simulink model "reactive_power_compensation"  (R2017b)
settings: Solver=VariableStepAuto  StartTime=0.0  StopTime=1  MaxStep=1e-4  RelTol=1e-3
undefined symbols (not defined in the file): magnitude
libraries: powerlib x15, powerlib_meascontrol x2
settings Model: Creator=Damla  LastModifiedBy=dagac

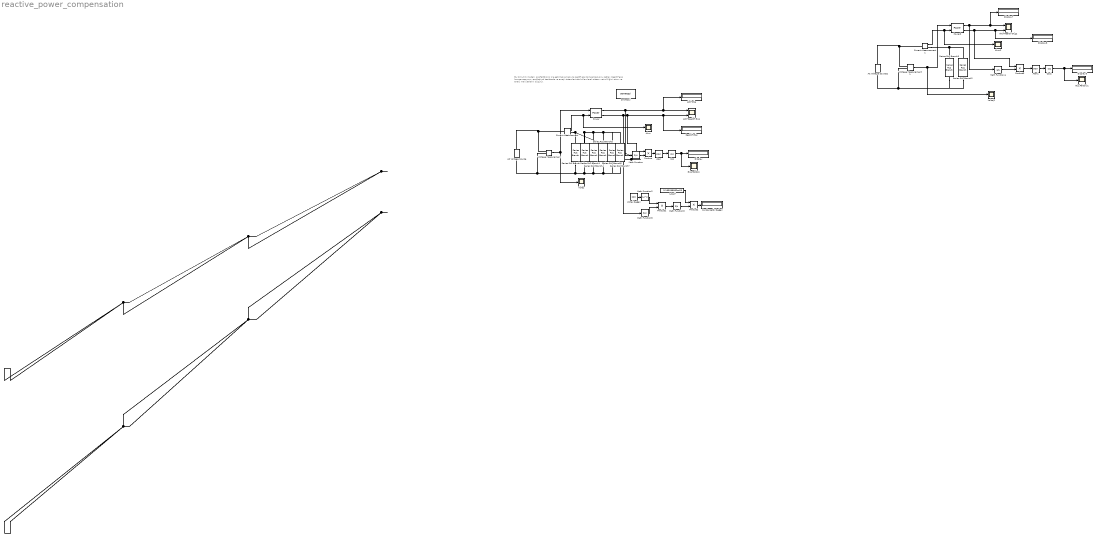
== system reactive_power_compensation ==
  note: Bu Simulink modeli, güç faktörünü 1'e getirmek amacıyla reaktif güç kompanzasyonu sağlar.
      | Reaktif güç kompanzasyonu, endüstriyel tesislerde ve enerji sistemlerinde kullanılarak
      | sistem verimliliğini artırır ve enerji maliyetlerini düşürür.
  1/2pif : Constant  Value=3.183098862e-03
  AC Voltage Source : powerlib/Electrical Sources/AC Voltage Source  Amplitude=220  Phase=0  Frequency=50  SampleTime=0  Measurements=None  BusType=swing  Pref=10e3  Qref=0  Qmin=-inf  Qmax=+inf
  AC Voltage Source2 : powerlib/Electrical Sources/AC Voltage Source  Amplitude=220  Phase=0  Frequency=50  SampleTime=0  Measurements=None  BusType=swing  Pref=10e3  Qref=0  Qmin=-inf  Qmax=+inf
  Aktif Güç : Display
  Aktif Reaktif Güç : Scope  NumInputPorts=2
  Aktif Reaktif Güç2 : Scope  NumInputPorts=2
  Akım : Scope
  Akım2 : Scope
  Atan : Trigonometry  Operator=atan
  Atan1 : Trigonometry  Operator=atan
  Cos : Trigonometry  Operator=cos
  Cos2 : Trigonometry  Operator=cos
  Current Measurement : powerlib/Measurements/Current Measurement  PhasorSimulation=off  OutputType=Complex  PSBequivalent=0
  Current Measurement1 : powerlib/Measurements/Current Measurement  PhasorSimulation=off  OutputType=Complex  PSBequivalent=0
  Display{,5,7..8} (4 alike) : Display
  Güç Faktörü : Scope
  Güç Faktörü1 : Scope
  Kondansatör Değeri : Display
  Math Function{,3..5} (4 alike) : Math  Operator=reciprocal  SaturateOnIntegerOverflow=on
  Math Function2 : Math  Operator=magnitude^2  SaturateOnIntegerOverflow=on
  Power : powerlib_meascontrol/Measurements/Power  Freq=50  Vinit=[1, 0]  Iinit=[1, 0]  Ts=0
      settings: SourceProductName=Simscape Power Systems
  Power2 : powerlib_meascontrol/Measurements/Power  Freq=50  Vinit=[1, 0]  Iinit=[1, 0]  Ts=0
      settings: SourceProductName=Simscape Power Systems
  Product{,1..3} (4 alike) : Product
  Reaktif Güç : Display
  Series RLC Branch : powerlib/Elements/Series RLC Branch  LConnTagsString=__new0  RConnTagsString=__new0  BranchType=RL  Resistance=12  Inductance=0.01  SetiL0=off  InitialCurrent=0  Capacitance=1e-6  Setx0=off  InitialVoltage=0  Measurements=None
  Series RLC Branch1 : powerlib/Elements/Series RLC Branch  LConnTagsString=__new0  RConnTagsString=__new0  BranchType=RC  Resistance=0.1  Inductance=0.01  SetiL0=off  InitialCurrent=0  Capacitance=3.25e-05  Setx0=off  InitialVoltage=0  Measurements=None
  Series RLC Branch2 : powerlib/Elements/Series RLC Branch  LConnTagsString=__new0  RConnTagsString=__new0  BranchType=RC  Resistance=0.1  Inductance=0.01  SetiL0=off  InitialCurrent=0  Capacitance=3.25e-05  Setx0=off  InitialVoltage=0  Measurements=None
  Series RLC Branch3 : powerlib/Elements/Series RLC Branch  LConnTagsString=__new0  RConnTagsString=__new0  BranchType=RL  Resistance=12  Inductance=0.01  SetiL0=off  InitialCurrent=0  Capacitance=1e-6  Setx0=off  InitialVoltage=0  Measurements=None
  Series RLC Branch4 : powerlib/Elements/Series RLC Branch  LConnTagsString=__new0  RConnTagsString=__new0  BranchType=RC  Resistance=0.1  Inductance=0.01  SetiL0=off  InitialCurrent=0  Capacitance=1.624e-05  Setx0=off  InitialVoltage=0  Measurements=None
  Series RLC Branch5 : powerlib/Elements/Series RLC Branch  LConnTagsString=__new0  RConnTagsString=__new0  BranchType=RC  Resistance=0.1  Inductance=0.01  SetiL0=off  InitialCurrent=0  Capacitance=8.124e-06  Setx0=off  InitialVoltage=0  Measurements=None
  Series RLC Branch6 : powerlib/Elements/Series RLC Branch  LConnTagsString=__new0  RConnTagsString=__new0  BranchType=RC  Resistance=0.1  Inductance=0.01  SetiL0=off  InitialCurrent=0  Capacitance=4.062e-06  Setx0=off  InitialVoltage=0  Measurements=None
  Series RLC Branch7 : powerlib/Elements/Series RLC Branch  LConnTagsString=__new0  RConnTagsString=__new0  BranchType=RC  Resistance=0.1  Inductance=0.01  SetiL0=off  InitialCurrent=0  Capacitance=2.032e-06  Setx0=off  InitialVoltage=0  Measurements=None
  Voltage Measurement : powerlib/Measurements/Voltage Measurement  PhasorSimulation=off  OutputType=Complex  PSBequivalent=0
  Voltage Measurement1 : powerlib/Measurements/Voltage Measurement  PhasorSimulation=off  OutputType=Complex  PSBequivalent=0
  Voltaj : Scope
  Voltaj Değeri : Constant  Value=220
  Voltaj2 : Scope
  powergui : powerlib/powergui  Priority=1  SimulationMode=Continuous  SampleTime=50e-6  frequency=60  Iterations=50  frequencyindice=50  Pbase=100e6  ErrMax=1e-4  UnitsV=kV  UnitsW=MW  buscounter=0  FunctionMessages=off  echomessages=off  EnableUseOfTLC=off  CurrentSourceSwitches=off  DisableSnubberDevices=off  DisableRonSwitches=off  DisableVfSwitches=off  DisplayEquations=off  SolverType=Tustin/Backward Euler (TBE)  Interpol=off  ExternalGateDelay=off  methode=off  Ts=100  x0status=blocks  SPID=on  SwTol=0  HookPort=off  RestoreLinks=warning  ResistiveCurrentMeasurement=off  Frange=[0:2:500]  Ylog=off  Xlog=on  ShowGrid=off  save=off  variable=ZData  structure=0  ZoomFFT=off  StartTime=0.0  cycles=1  DisplayStyle=1  fundamental=60  FreqAxis=off  MaxFrequency=1000  frequencyindicesteady=1  RmsSteady=1  display=off
  wires:
  Cos/1 -> Display/1, Güç Faktörü/1
  Atan/1 -> Cos/1
  Current Measurement/1 -> Power/2, Akım/1  "Akım"
  Power/1 -> Math Function/1, Aktif Reaktif Güç/1, Aktif Güç/1  "Aktif Güç"
  Product/1 -> Atan/1
  Math Function/1 -> Product/2
  Power/2 -> Math Function5/1, Aktif Reaktif Güç/2, Reaktif Güç/1, Product/1  "Reaktif Güç"
  Voltage Measurement/1 -> Power/1, Voltaj/1  "Voltaj"
  Cos2/1 -> Güç Faktörü1/1, Display5/1
  Current Measurement1/1 -> Power2/2, Akım2/1
  Voltage Measurement1/1 -> Power2/1, Voltaj2/1
  Atan1/1 -> Cos2/1
  Math Function4/1 -> Product3/2
  Product3/1 -> Atan1/1
  Power2/1 -> Math Function4/1, Display7/1, Aktif Reaktif Güç2/1  "Aktif Güç"
  Power2/2 -> Display8/1, Aktif Reaktif Güç2/2, Product3/1  "Reaktif Güç"
  Math Function2/1 -> Product1/1
  Product1/1 -> Math Function3/1
  Math Function3/1 -> Product2/2
  1/2pif/1 -> Product2/1
  Product2/1 -> Kondansatör Değeri/1
  Math Function5/1 -> Product1/2
  Voltaj Değeri/1 -> Math Function2/1
  connections:
  Voltage Measurement/LConn2 -- Series RLC Branch7/RConn1 -- Series RLC Branch6/RConn1 -- Series RLC Branch5/RConn1 -- Series RLC Branch4/RConn1 -- Series RLC Branch1/RConn1 -- Series RLC Branch/RConn1 -- AC Voltage Source/LConn1
  Current Measurement/LConn1 -- AC Voltage Source/RConn1 -- Voltage Measurement/LConn1
  Current Measurement/RConn1 -- Series RLC Branch7/LConn1 -- Series RLC Branch6/LConn1 -- Series RLC Branch5/LConn1 -- Series RLC Branch4/LConn1 -- Series RLC Branch1/LConn1 -- Series RLC Branch/LConn1
  Voltage Measurement1/LConn2 -- Series RLC Branch2/RConn1 -- Series RLC Branch3/RConn1 -- AC Voltage Source2/LConn1
  Current Measurement1/LConn1 -- AC Voltage Source2/RConn1 -- Voltage Measurement1/LConn1
  Current Measurement1/RConn1 -- Series RLC Branch2/LConn1 -- Series RLC Branch3/LConn1
  ?
  ?
